simulink model "Part1_sim"  (R2024b)
settings: Solver=ode23tb  StartTime=0.0  StopTime=25  FixedStep=1  RelTol=1e-3
settings Model: Creator=juanq  LastModifiedBy=juanq

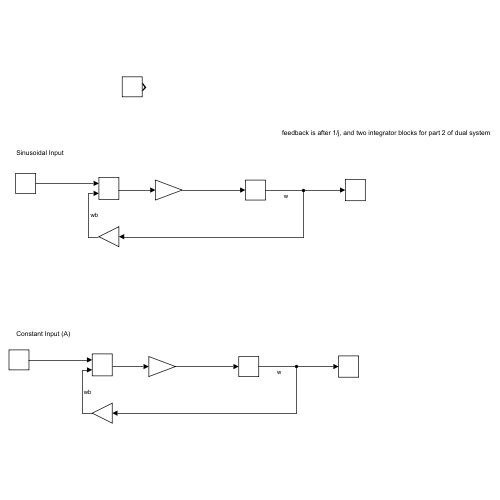
[thumbnail: Simulink's stored preview of the top-level diagram]
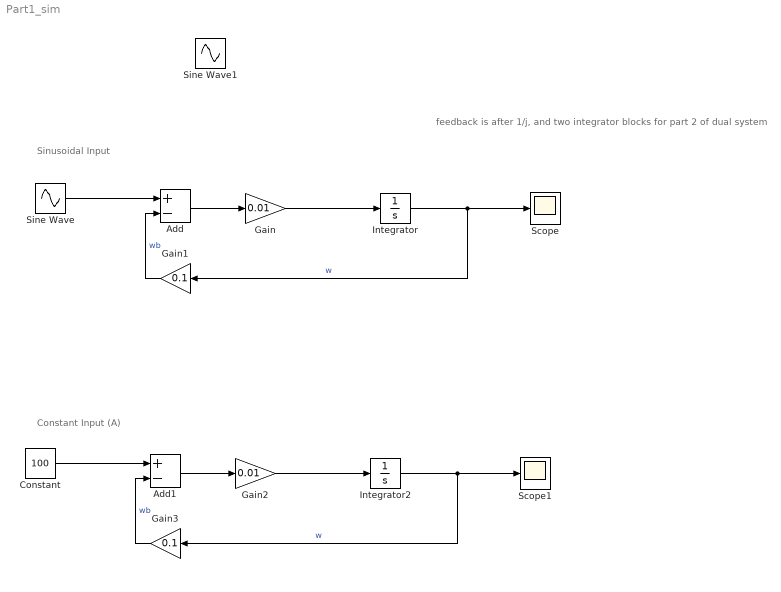
== system Part1_sim ==
  note: Sinusoidal Input
  note: Constant Input (A)
  note: feedback is after 1/j, and two integrator blocks for part 2 of dual system
  Add : Sum  Inputs=+-
  Add1 : Sum  Inputs=+-
  Constant : Constant  Value=100
  Gain : Gain  Gain=0.01
  Gain1 : Gain  Gain=0.1
  Gain2 : Gain  Gain=0.01
  Gain3 : Gain  Gain=0.1
  Integrator : Integrator
  Integrator2 : Integrator  IgnoreLimit=on
  Scope : Scope
  Scope1 : Scope
  Sine Wave : Sin  Frequency=100  SampleTime=0
  Sine Wave1 : Sin  SampleTime=0
  wires:
  Sine Wave/1 -> Add/1
  Gain1/1 -> Add/2  "wb"
  Add/1 -> Gain/1
  Gain/1 -> Integrator/1
  Integrator/1 -> Scope/1, Gain1/1  "w"
  Gain3/1 -> Add1/2  "wb"
  Constant/1 -> Add1/1
  Add1/1 -> Gain2/1
  Integrator2/1 -> Scope1/1, Gain3/1  "w"
  Gain2/1 -> Integrator2/1
